simulink model "slexVariantSubsystemsWithParSim_"  (R2023b)
settings: Solver=FixedStepAuto  StartTime=0.0  StopTime=100000  RelTol=1e-3  EnableMultiTasking=on
PreLoadFcn:
  | VSS_MODE = Simulink.Parameter(int32(1));
  | VSS_MODE.StorageClass = 'ExportedGlobal';
StartFcn:
  | tic;
StopFcn:
  | toc
Description:
  | Variant Subsystems
  | 
  | This model illustrates Simulink(R) variant subsystems. Variant subsystems let
  | you provide multiple implementations to a subsystem where only one
  | implementation is active during simulation. You can programmatically swap out
  | the active implementation and replace it with one of the other implementations
  | without modifying the model.
settings Model: FPTRunName=Active  SimulationMode=rapid-accelerator  Creator=The MathWorks, Inc.  LastModifiedBy=gschrabe
settings SolverCC: AlgebraicLoopSolver=TrustRegion
settings DataIOCC: LimitDataPoints=on
settings OptimizationCC: DefaultParameterBehavior=Inlined  EnhancedBackFolding=on  PassReuseOutputArgsAs=Individual arguments  ExpressionDepthLimit=2147483647  ZeroExternalMemoryAtStartup=off  ZeroInternalMemoryAtStartup=off  OptimizeBlockOrder=speed  DifferentSizesBufferReuse=on  OptimizationCustomize=off  EfficientTunableParamExpr=on
settings DebuggingCC: SolverPrmCheckMsg=warning  ParameterTunabilityLossMsg=error  FcnCallInpInsideContextMsg=warning  UnconnectedInputMsg=warning  UnconnectedOutputMsg=warning  UnconnectedLineMsg=warning  StateNameClashWarn=warning  SFUnexpectedBacktrackingDiag=warning  SFNoUnconditionalDefaultTransitionDiag=warning  SFExecutionAtInitializationDiag=none  ArithmeticOperatorsInVariantConditions=warning
settings HardwareCC: ProdBitPerPointer=32  ProdBitPerSizeT=32  ProdBitPerPtrDiffT=32  ProdLargestAtomicFloat=None  ProdIntDivRoundTo=Undefined  ProdEndianess=Unspecified  ProdWordSize=32  ProdHWDeviceType=32-bit Generic
settings ModelReferenceCC: EnableRefExpFcnMdlSchedulingChecks=on  PropagateSignalLabelsOutOfModel=off
settings SFSimCC: SimUseLocalCustomCode=off  MATLABDynamicMemAlloc=off
settings RTWCC: Description=Embedded Coder  SystemTargetFile=ert.tlc  TemplateMakefile=ert_default_tmf  RTWUseLocalCustomCode=off  DLArmComputeVersion=19.05
settings CodeAppCC: ForceParamTrailComments=on  IgnoreCustomStorageClasses=off  OperatorAnnotations=on  SimulinkDataObjDesc=on  SFDataObjDesc=on  InsertBlockDesc=on
settings ERTTargetCC: GenerateSampleERTMain=on  InlinedParameterPlacement=NonHierarchical  ERTCustomFileTemplate=example_file_process.tlc
settings ConfigComp: CovMetricSettings=dw  CovSaveCumulativeToWorkspaceVar=on  CovSaveSingleToWorkspaceVar=on  CovExternalEMLEnable=off  CovSFcnEnable=off

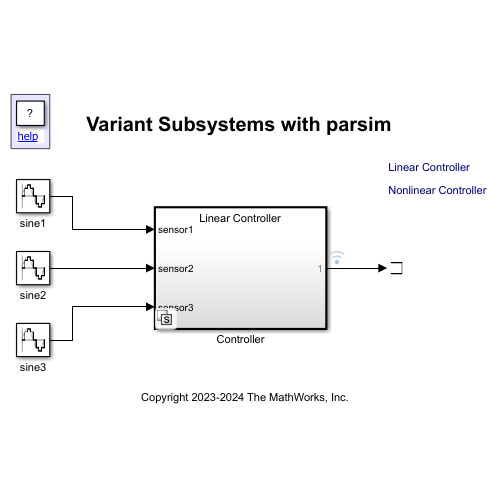
[thumbnail: Simulink's stored preview of the top-level diagram]
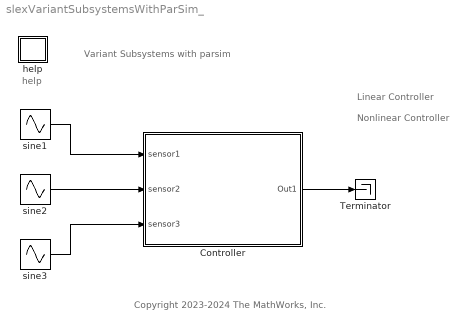
== system slexVariantSubsystemsWithParSim_ ==
  note: Nonlinear Controller
  note: Linear Controller
  note: Copyright 2023-2024 The MathWorks, Inc.
  note: Variant Subsystems with parsim
  note: help
  Controller : Subsystem  Variant=on  VariantActivationTime=startup
  Terminator : Terminator
  help : Subsystem
      mask Display: disp('?')
  sine1 : Sin  Amplitude=.1  Frequency=pi/3  SampleTime=.01
  sine2 : Sin  Amplitude=2  SampleTime=.01
  sine3 : Sin  Amplitude=.3  Frequency=pi/6  SampleTime=.01
  wires:
  sine2/1 -> Controller/2(sensor2)
  sine1/1 -> Controller/1(sensor1)
  sine3/1 -> Controller/3(sensor3)
  Controller/1(Out1) -> Terminator/1

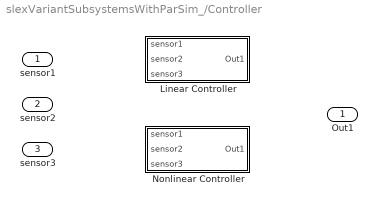
== system slexVariantSubsystemsWithParSim_/Controller ==
  sensor1 : Inport
  sensor2 : Inport  Port=2
  sensor3 : Inport  Port=3
  Linear Controller : Subsystem  TreatAsAtomicUnit=on  VariantControl=VSS_MODE==1
  Nonlinear Controller : Subsystem  TreatAsAtomicUnit=on  VariantControl=VSS_MODE==2
  Out1 : Outport  VectorParamsAs1DForOutWhenUnconnected=off

== system slexVariantSubsystemsWithParSim_/help ==
  note: This example illustrates how Variant Subsystem with startup activation can be simulated using parsim. Open slexVariantSubsystemsWithParSim_script.m to run each steps.
      | Step 1
      | % setup the active variant selection for each variant choice
      | % and set the number of simulation run equal to the variant selections
      | mdl = 'slexVariantSubsystemsWithParSim' ;
      | numSims = 2;
      | varControl = [1,2];
      |
      | Step 2
      | % create the SimulationInput object for each simulation run
      | % and set the Variant Control value for each run
      | in(1:numSims) = Simulink.SimulationInput(mdl);
      | for idx = 1:numSims
      | in(idx) = in(idx).setModelParameter( 'SimulationMode' , 'rapid' , ...
      | 'RapidAcceleratorUpToDateCheck' , 'on' , ...
      | 'SaveTime' , 'on' , ...
      | 'SaveOutput' , 'on' );
      | in(idx) = in(idx).setVariable( 'VSS_MODE' ,varControl(idx));
      | end
      |
      | Step 3
      | % Using parsim Simulate the model in parallel for each variant control value
      | out = parsim(in, 'ShowProgress' , 'on' );
      |
      | Step 4
      | % Now plot the output values each run
      | for i = 1:numSims
      | simOut = out(i);
      | t = simOut.tout;
      | y = simOut.yout;
      | plot(t, y)
      | hold all
      | end

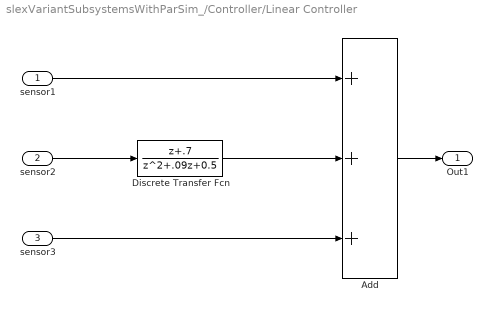
== system slexVariantSubsystemsWithParSim_/Controller/Linear Controller ==
  sensor1 : Inport
  sensor2 : Inport  Port=2
  sensor3 : Inport  Port=3
  Add : Sum  Inputs=+++
  Discrete Transfer Fcn : DiscreteTransferFcn  Numerator=[1 .7]  Denominator=[1 .09 0.5]  SampleTime=.01
  Out1 : Outport  VectorParamsAs1DForOutWhenUnconnected=off
  wires:
  sensor2/1 -> Discrete Transfer Fcn/1
  Discrete Transfer Fcn/1 -> Add/2
  sensor3/1 -> Add/3
  sensor1/1 -> Add/1
  Add/1 -> Out1/1

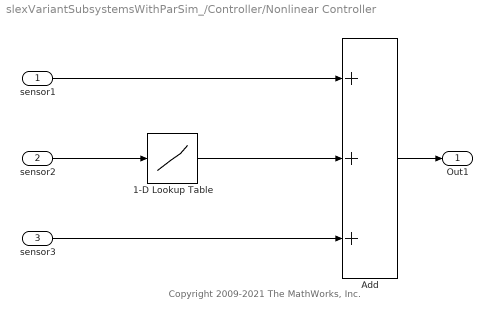
== system slexVariantSubsystemsWithParSim_/Controller/Nonlinear Controller ==
  note: Copyright 2009-2021 The MathWorks, Inc.
  sensor1 : Inport
  sensor2 : Inport  Port=2
  sensor3 : Inport  Port=3
  1-D Lookup Table : Lookup_n-D  NumberOfTableDimensions=1  BreakpointsForDimension1=[-5:5]  Table=tanh([-5:5])
  Add : Sum  Inputs=+++
  Out1 : Outport  VectorParamsAs1DForOutWhenUnconnected=off
  wires:
  sensor2/1 -> 1-D Lookup Table/1
  1-D Lookup Table/1 -> Add/2
  sensor3/1 -> Add/3
  sensor1/1 -> Add/1
  Add/1 -> Out1/1
